simulink model "FactorialStateFlow"  (R2018b)
settings: Solver=FixedStepDiscrete  StartTime=0.0  StopTime=10.0  RelTol=1e-3
settings Model: Creator=dahroug  LastModifiedBy=dahroug
settings OptimizationCC: DefaultParameterBehavior=Inlined  EnhancedBackFolding=on  PassReuseOutputArgsAs=Individual arguments  OptimizeBlockOrder=speed  DifferentSizesBufferReuse=on  OptimizationCustomize=off
settings DebuggingCC: UnderspecifiedInitializationDetection=Classic  MergeDetectMultiDrivingBlocksExec=none  ParameterTunabilityLossMsg=error
settings ModelReferenceCC: PropagateSignalLabelsOutOfModel=off
settings SFSimCC: MATLABDynamicMemAlloc=off
settings RTWCC: SystemTargetFile=ert.tlc  GenCodeOnly=on  TemplateMakefile=ert_default_tmf  GenerateReport=on  IncludeHyperlinkInReport=on  LaunchReport=on  GenerateTraceInfo=on  GenerateTraceReport=on  GenerateTraceReportSl=on  GenerateTraceReportSf=on  GenerateTraceReportEml=on
settings CodeAppCC: ForceParamTrailComments=on  IgnoreCustomStorageClasses=off  OperatorAnnotations=on  SimulinkDataObjDesc=on  SFDataObjDesc=on  InsertBlockDesc=on
settings ERTTargetCC: TargetLangStandard=C99 (ISO)  GenerateSampleERTMain=on  InlinedParameterPlacement=NonHierarchical  ERTCustomFileTemplate=example_file_process.tlc

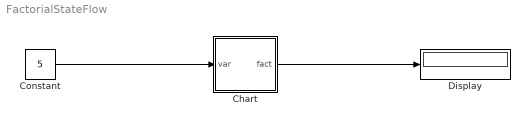
== system FactorialStateFlow ==
  Chart : Stateflow chart  TreatAsAtomicUnit=on
  Constant : Constant  Value=5  OutDataTypeStr=uint8
  Display : Display
  wires:
  Constant/1 -> Chart/1(var)
  Chart/1(fact) -> Display/1

== stateflow chart FactorialStateFlow/Chart ==
  (default) -> (junction 2)
  (junction 1) -> (junction 9) [order 1] : [counter>1]
  (junction 2) -> (junction 1) : {fact=1; counter=var;}
  (junction 9) -> (junction 13) : {fact=fact*counter;}
  (junction 13) -> (junction 1) : {counter=counter-1;}
  (junction 1) -> (junction 11) [order 2]
  data: var input uint8; fact output uint8; counter local uint8
